simulink model "SwcCELCmgrTest"  (R2016a)
settings: Solver=VariableStepDiscrete  StartTime=0.0  StopTime=10  RelTol=1e-3
undefined symbols (not defined in the file): sigbuilder_block
libraries: CELCmgrLogicLib x1
settings Model: Creator=uidp6624  LastModifiedBy=uidp6624

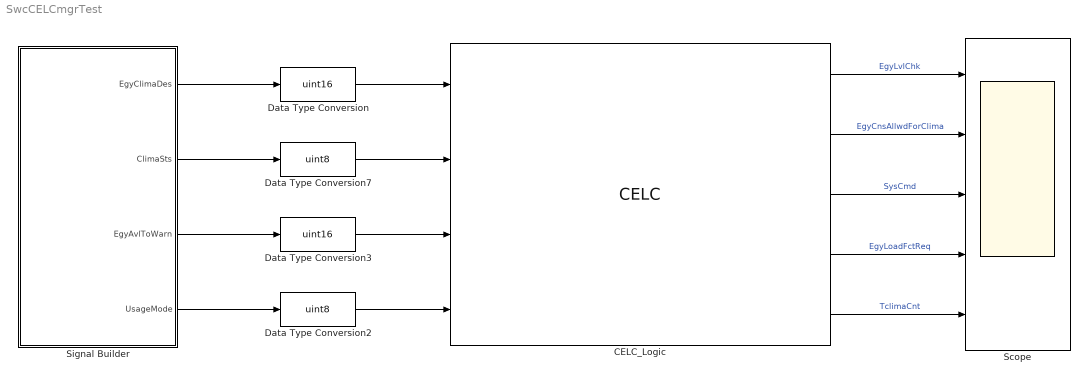
== system SwcCELCmgrTest ==
  CELC_Logic : CELCmgrLogicLib/CELC
  Data Type Conversion : DataTypeConversion  OutDataTypeStr=uint16
  Data Type Conversion2 : DataTypeConversion  OutDataTypeStr=uint8
  Data Type Conversion3 : DataTypeConversion  OutDataTypeStr=uint16
  Data Type Conversion7 : DataTypeConversion  OutDataTypeStr=uint8
  Scope : Scope  NumInputPorts=5
  Signal Builder : Subsystem  Tag=STV Subsys  LoadFcn=sigbuilder_block('load');  StartFcn=sigbuilder_block('start');  StopFcn=sigbuilder_block('stop');  ClipboardFcn=sigbuilder_block('clipboard');  mask(Sigbuilder block){}
      mask help: Simulink:masks:SigbuilderBlock_MD
      mask init:
      | if ~strcmp(get_param(bdroot(gcbh),'SimulationStatus'),'stopped') tuvar = sigbuilder_block('maskInit'); end
      settings: CopyFcn=sigbuilder_block('copy');  DeleteFcn=sigbuilder_block('delete');  ModelCloseFcn=sigbuilder_block('modelClose');  PreSaveFcn=sigbuilder_block('preSave');  PauseFcn=sigbuilder_block('pause');  ContinueFcn=sigbuilder_block('continue');  NameChangeFcn=sigbuilder_block('namechange');  OpenFcn=sigbuilder_block('open',[1152 0 1152 592.8 ]);  CloseFcn=sigbuilder_block('close');
      mask Display: plot(0, 0, 100, 100,[2, 2, 32, 32, 2], [68, 8, 8, 68, 68],[32, 2], [38, 38], [32, 19, 2],[53, 60, 44], [32, 17, 17, 2],[16, 16, 31, 31]);txt = getActiveGroup(gcbh);text(2, 100, txt,'verticalAlignment', 'top');
  wires:
  Signal Builder/1(EgyClimaDes) -> Data Type Conversion/1
  CELC_Logic/1 -> Scope/1  "EgyLvlChk"
  Data Type Conversion/1 -> CELC_Logic/1
  Data Type Conversion2/1 -> CELC_Logic/4
  CELC_Logic/2 -> Scope/2  "EgyCnsAllwdForClima"
  Signal Builder/2(ClimaSts) -> Data Type Conversion7/1
  Data Type Conversion7/1 -> CELC_Logic/2
  Signal Builder/3(EgyAvlToWarn) -> Data Type Conversion3/1
  Data Type Conversion3/1 -> CELC_Logic/3
  CELC_Logic/3 -> Scope/3  "SysCmd"
  CELC_Logic/4 -> Scope/4  "EgyLoadFctReq"
  CELC_Logic/5 -> Scope/5  "TclimaCnt"
  Signal Builder/4(UsageMode) -> Data Type Conversion2/1

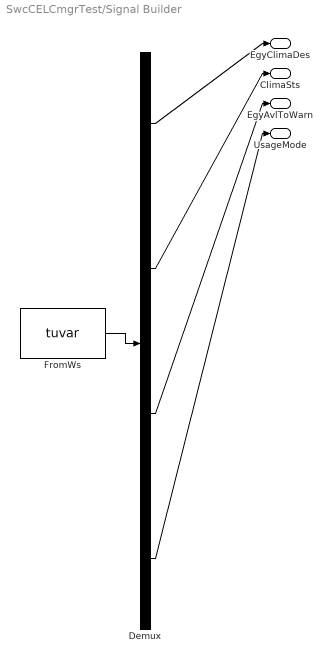
== system SwcCELCmgrTest/Signal Builder ==
  Demux : Demux  Tag=STV Demux
  FromWs : FromWorkspace  Tag=STV FromWs  VariableName=tuvar  SampleTime=0
      SigBuilderData=|
      | common.afterFinalStr = 'Extrapolate'
      | common.sampleTime = 0
      | dataSet(1).timeRange = [0 10]
      | dataSet(1).name = 'CELCTestCase1:OFF-->CHECK'
      | dataSet(2).timeRange = [0 10]
      | dataSet(2).name = 'CELCTestCase2:CHECK-->EGY_CALC-->ACTIVE_USAGRMODE'
      | dataSet(3).timeRange = [0 10]
      | dataSet(3).name = 'CELCTestCase3:CHECK-->EGY_CALC-->ACTUATOR_OFF'
      | dataSet(4).timeRange = [0 10]
      | dataSet(4).name = 'CELCTestCase4:ACTIVE_USAGRMODE-->ACTUATOR_ON'
      | dataSet(5).timeRange = [0 10]
      | dataSet(5).name = 'CELCTestCase5:ACTUATOR_ON-->ACTUATOR_OFF'
      | dataSet(6).timeRange = [0 10]
      | dataSet(6).name = 'CELCTestCase6:ACTUATOR_ON-->ACTUATOR_OFF'
      | sbobj.Groups(1).Name = 'CELCTestCase1:OFF-->CHECK'
      | sbobj.Groups(1).Signals(1).Name = 'EgyClimaDes'
      | sbobj.Groups(1).Signals(1).XData = [0 2 2 6 10]
      | sbobj.Groups(1).Signals(1).YData = [0 0 1 1 1]
      | sbobj.Groups(1).Signals(2).Name = 'ClimaSts'
      | sbobj.Groups(1).Signals(2).XData = [0 4 6 10]
      | sbobj.Groups(1).Signals(2).YData = [0 0 0 0]
      | sbobj.Groups(1).Signals(3).Name = 'EgyAvlToWarn'
      | sbobj.Groups(1).Signals(3).XData = [0 2.022 5.009 10]
      | sbobj.Groups(1).Signals(3).YData = [0 0 0 0]
      | sbobj.Groups(1).Signals(4).Name = 'UsageMode'
      | sbobj.Groups(1).Signals(4).XData = [0 3.01 9.45 10]
      | sbobj.Groups(1).Signals(4).YData = [0 0 0 0]
      | sbobj.Groups(2).Name = 'CELCTestCase2:CHECK-->EGY_CALC-->ACTIVE_USAGRMODE'
      | sbobj.Groups(2).Signals(1).Name = 'EgyClimaDes'
      | sbobj.Groups(2).Signals(1).XData = [0 2 2 6 10]
      | sbobj.Groups(2).Signals(1).YData = [0 0 1 1 1]
      | sbobj.Groups(2).Signals(2).Name = 'ClimaSts'
      | sbobj.Groups(2).Signals(2).XData = [0 4 6 10]
      | sbobj.Groups(2).Signals(2).YData = [0 0 0 0]
      | sbobj.Groups(2).Signals(3).Name = 'EgyAvlToWarn'
      | sbobj.Groups(2).Signals(3).XData = [0 3.01 3.01 5.009 5.009 10]
      | sbobj.Groups(2).Signals(3).YData = [0 0 1 1 0.99 0.99]
      | sbobj.Groups(2).Signals(4).Name = 'UsageMode'
      | sbobj.Groups(2).Signals(4).XData = [0 3.99 9.45 10]
      | sbobj.Groups(2).Signals(4).YData = [0 0 0 0]
      | sbobj.Groups(3).Name = 'CELCTestCase3:CHECK-->EGY_CALC-->ACTUATOR_OFF'
      | sbobj.Groups(3).Signals(1).Name = 'EgyClimaDes'
      | sbobj.Groups(3).Signals(1).XData = [0 2 2 3 3 10]
      | sbobj.Groups(3).Signals(1).YData = [0 0 1 1 0 0]
      | sbobj.Groups(3).Signals(2).Name = 'ClimaSts'
      | sbobj.Groups(3).Signals(2).XData = [0 2 2 6.33 10]
      | sbobj.Groups(3).Signals(2).YData = [0 0 1 1 1]
      | sbobj.Groups(3).Signals(3).Name = 'EgyAvlToWarn'
      | sbobj.Groups(3).Signals(3).XData = [0 3 3 5.009 10]
      | sbobj.Groups(3).Signals(3).YData = [0 0 1 1 1]
      | sbobj.Groups(3).Signals(4).Name = 'UsageMode'
      | sbobj.Groups(3).Signals(4).XData = [0 3.01 9.45 10]
      | sbobj.Groups(3).Signals(4).YData = [0 0 0 0]
      | sbobj.Groups(4).Name = 'CELCTestCase4:ACTIVE_USAGRMODE-->ACTUATOR_ON'
      | sbobj.Groups(4).Signals(1).Name = 'EgyClimaDes'
      | sbobj.Groups(4).Signals(1).XData = [0 2 2 6 10]
      | sbobj.Groups(4).Signals(1).YData = [0 0 1 1 1]
      | sbobj.Groups(4).Signals(2).Name = 'ClimaSts'
      | sbobj.Groups(4).Signals(2).XData = [0 4 6 10]
      | sbobj.Groups(4).Signals(2).YData = [0 0 0 0]
      | sbobj.Groups(4).Signals(3).Name = 'EgyAvlToWarn'
      | sbobj.Groups(4).Signals(3).XData = [0 3.01 3.01 5.009 5.009 10]
      | sbobj.Groups(4).Signals(3).YData = [0 0 1 1 0.99 0.99]
      | sbobj.Groups(4).Signals(4).Name = 'UsageMode'
      | sbobj.Groups(4).Signals(4).XData = [0 3.99 3.99 9.45 10]
      | sbobj.Groups(4).Signals(4).YData = [0 0 1 1 1]
      | sbobj.Groups(5).Name = 'CELCTestCase5:ACTUATOR_ON-->ACTUATOR_OFF'
      | sbobj.Groups(5).Signals(1).Name = 'EgyClimaDes'
      | sbobj.Groups(5).Signals(1).XData = [0 2 2 5.01 5.01 10]
      | sbobj.Groups(5).Signals(1).YData = [0 0 1 1 0 0]
      | sbobj.Groups(5).Signals(2).Name = 'ClimaSts'
      | sbobj.Groups(5).Signals(2).XData = [0 4 6 10]
      | sbobj.Groups(5).Signals(2).YData = [0 0 0 0]
      | sbobj.Groups(5).Signals(3).Name = 'EgyAvlToWarn'
      | sbobj.Groups(5).Signals(3).XData = [0 3.01 3.01 5.009 5.009 10]
      | sbobj.Groups(5).Signals(3).YData = [0 0 1 1 0.99 0.99]
      | sbobj.Groups(5).Signals(4).Name = 'UsageMode'
      | sbobj.Groups(5).Signals(4).XData = [0 3.99 3.99 5.01 5.01 10]
      | sbobj.Groups(5).Signals(4).YData = [0 0 1 1 0 0]
      | sbobj.Groups(6).Name = 'CELCTestCase6:ACTUATOR_ON-->ACTUATOR_OFF'
      | sbobj.Groups(6).Signals(1).Name = 'EgyClimaDes'
      | sbobj.Groups(6).Signals(1).XData = [0 2 2 5.01 5.01 10]
      | sbobj.Groups(6).Signals(1).YData = [0 0 1 1 0 0]
      | sbobj.Groups(6).Signals(2).Name = 'ClimaSts'
      | sbobj.Groups(6).Signals(2).XData = [0 4 6 10]
      | sbobj.Groups(6).Signals(2).YData = [0 0 0 0]
      | sbobj.Groups(6).Signals(3).Name = 'EgyAvlToWarn'
      | sbobj.Groups(6).Signals(3).XData = [0 3.01 3.01 5.009 5.009 10]
      | sbobj.Groups(6).Signals(3).YData = [0 0 1 1 0.99 0.99]
      | sbobj.Groups(6).Signals(4).Name = 'UsageMode'
      | sbobj.Groups(6).Signals(4).XData = [0 3.99 3.99 5.01 10]
      | sbobj.Groups(6).Signals(4).YData = [0 0 1 1 1]
  EgyClimaDes : Outport  Tag=STV Outport
  ClimaSts : Outport  Tag=STV Outport  Port=2
  EgyAvlToWarn : Outport  Tag=STV Outport  Port=3
  UsageMode : Outport  Tag=STV Outport  Port=4
  wires:
  FromWs/1 -> Demux/1
  Demux/1 -> EgyClimaDes/1
  Demux/2 -> ClimaSts/1
  Demux/3 -> EgyAvlToWarn/1
  Demux/4 -> UsageMode/1
